simulink model "ADAS_System"  (R2025b)
settings: Solver=FixedStepAuto  StartTime=0.0  StopTime=15  FixedStep=0.01  RelTol=1e-3
values from neighbouring files (symbols this model uses):
  d_init = 160    [init_ADAS.m]
  fs = 100    [init_ADAS.m]
  v_ego = 40    [init_ADAS.m]
  v_lead = 25    [init_ADAS.m]
libraries: simulink x2
settings Model: Creator=szymo  LastModifiedBy=Janek

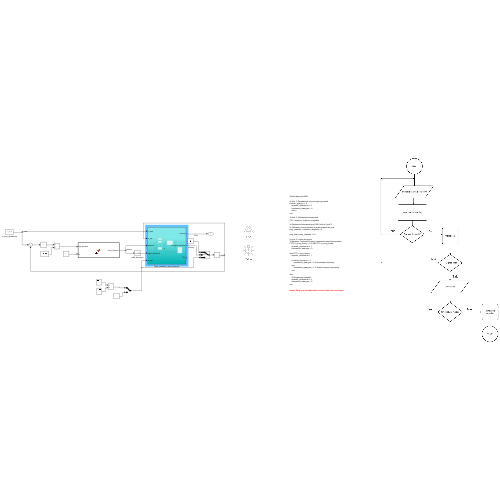
[thumbnail: Simulink's stored preview of the top-level diagram]
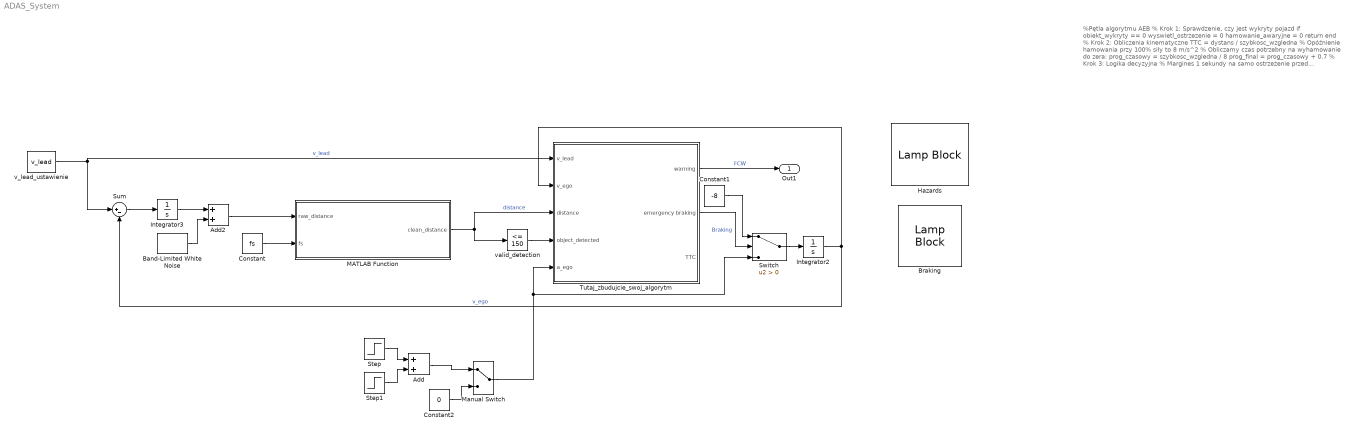
== system ADAS_System ==
  note: %Pętla algorytmu AEB
      |
      | % Krok 1: Sprawdzenie, czy jest wykryty pojazd
      | if obiekt_wykryty == 0
      | wyswietl_ostrzezenie = 0
      | hamowanie_awaryjne = 0
      | return
      | end
      |
      | % Krok 2: Obliczenia kinematyczne
      | TTC = dystans / szybkosc_wzgledna
      |
      | % Opóźnienie hamowania przy 100% siły to 8 m/s^2
      | % Obliczamy czas potrzebny na wyhamowanie do zera:
      | prog_czasowy = szybkosc_wzgledna / 8
      |
      | prog_final = prog_czasowy + 0.7
      |
      | % Krok 3: Logika decyzyjna
      | % Margines 1 sekundy na samo ostrzeżenie przed hamowaniem
      | if TTC < (prog_finalny + 1.0) AND TTC >= prog_finalny
      | wyswietl_ostrzezenie = 1
      | hamowanie_awaryjne = 0
      |
      | elseif TTC < prog_finalny
      | wyswietl_ostrzezenie = 1
      |
      | if reakcja_kierowcy == 1
      | hamowanie_awaryjne = 0 % Hamowanie kierowcy
      | else
      | hamowanie_awaryjne = 1 % System hamuje z pełną siłą
      | end
      |
      | else
      | % Bezpieczna odległość
      | wyswietl_ostrzezenie = 0
      | hamowanie_awaryjne = 0
      | end
      |
      | Uwagi: Zmiany w pseudokodzie oznaczać kolorem czerwonym
  Add : Sum
  Add2 : Sum
  Band-Limited White Noise : simulink/Sources/Band-Limited White Noise  Cov=[0.1]  Ts=0.1  seed=[23341]
  Braking : LampBlock  LabelPosition=Bottom  DefaultColor=[192.0, 192.0, 192.0]  Icon=ExteriorBulbFailure
  Constant : Constant  Value=fs
  Constant1 : Constant  Value=-8
  Constant2 : Constant  Value=0
  Hazards : LampBlock  LabelPosition=Bottom  DefaultColor=[192.0, 192.0, 192.0]  Icon=Hazards
  Integrator2 : Integrator  InitialCondition=v_ego
  Integrator3 : Integrator  InitialCondition=d_init
  MATLAB Function : MATLAB Function  TreatAsAtomicUnit=on
  Manual Switch : ManualSwitch
  Step : Step  Time=8.0  After=-8  SampleTime=0
  Step1 : Step  Time=8.1  After=3  SampleTime=0
  Sum : Sum  Inputs=|+-
  Switch : Switch  Criteria=u2 > Threshold  SaturateOnIntegerOverflow=off  InputSameDT=off
  Tutaj_zbudujcie_swoj_algorytm : Subsystem
  v_lead_ustawienie : Constant  Value=v_lead
  valid_detection : simulink/Logic and Bit Operations/Compare To Constant  relop=<=  const=150  OutDataTypeStr=boolean
  Out1 : Outport
  wires:
  Band-Limited White Noise/1 -> Add2/2
  Add2/1 -> MATLAB Function/1(raw_distance)
  Constant/1 -> MATLAB Function/2(fs)
  Switch/1 -> Integrator2/1
  Integrator2/1 -> Tutaj_zbudujcie_swoj_algorytm/2(v_ego), Sum/2  "v_ego"
  v_lead_ustawienie/1 -> Sum/1, Tutaj_zbudujcie_swoj_algorytm/1(v_lead)  "v_lead"
  Sum/1 -> Integrator3/1
  Integrator3/1 -> Add2/1
  MATLAB Function/1(clean_distance) -> valid_detection/1, Tutaj_zbudujcie_swoj_algorytm/3(distance)  "distance"
  valid_detection/1 -> Tutaj_zbudujcie_swoj_algorytm/4(object_detected)
  Tutaj_zbudujcie_swoj_algorytm/1(warning) -> Out1/1  "FCW"
  Manual Switch/1 -> Tutaj_zbudujcie_swoj_algorytm/5(a_ego), Switch/3
  Constant1/1 -> Switch/1
  Tutaj_zbudujcie_swoj_algorytm/2(emergency braking) -> Switch/2  "Braking"
  Step/1 -> Add/1
  Step1/1 -> Add/2
  Add/1 -> Manual Switch/1
  Constant2/1 -> Manual Switch/2

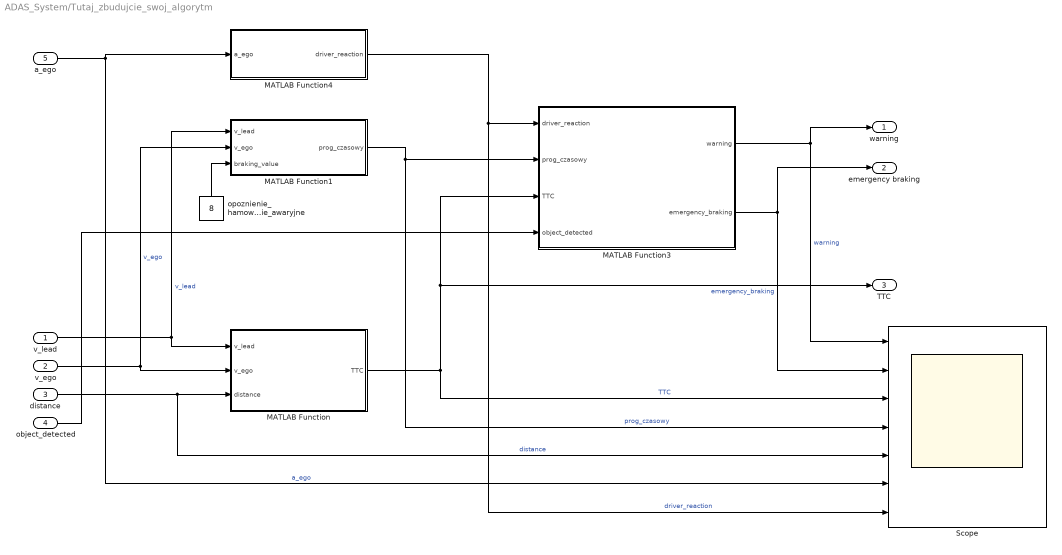
== system ADAS_System/Tutaj_zbudujcie_swoj_algorytm ==
  v_lead : Inport
  v_ego : Inport  Port=2
  distance : Inport  Port=3
  object_detected : Inport  Port=4
  a_ego : Inport  Port=5
  MATLAB Function : MATLAB Function  TreatAsAtomicUnit=on
  MATLAB Function1 : MATLAB Function  TreatAsAtomicUnit=on
  MATLAB Function3 : MATLAB Function  TreatAsAtomicUnit=on
  MATLAB Function4 : MATLAB Function  TreatAsAtomicUnit=on
  Scope : Scope  NumInputPorts=7
      settings: ActiveDisplayYMinimum=146.60609741255024  ActiveDisplayYMaximum=156.61068554348952
  opoznienie_hamowanie_awaryjne : Constant  Value=8
  warning : Outport
  emergency braking : Outport  Port=2
  "TTC " : Outport  Port=3
  wires:
  object_detected/1 -> MATLAB Function3/4(object_detected)
  MATLAB Function3/2(emergency_braking) -> emergency braking/1, Scope/2  "emergency_braking"
  MATLAB Function1/1(prog_czasowy) -> Scope/4, MATLAB Function3/2(prog_czasowy)  "prog_czasowy"
  MATLAB Function/1(TTC) -> MATLAB Function3/3(TTC), "TTC "/1, Scope/3  "TTC"
  v_lead/1 -> MATLAB Function1/1(v_lead), MATLAB Function/1(v_lead)  "v_lead"
  opoznienie_hamowanie_awaryjne/1 -> MATLAB Function1/3(braking_value)
  MATLAB Function3/1(warning) -> warning/1, Scope/1  "warning"
  v_ego/1 -> MATLAB Function1/2(v_ego), MATLAB Function/2(v_ego)  "v_ego"
  distance/1 -> MATLAB Function/3(distance), Scope/5  "distance"
  a_ego/1 -> Scope/6, MATLAB Function4/1(a_ego)  "a_ego"
  MATLAB Function4/1(driver_reaction) -> Scope/7, MATLAB Function3/1(driver_reaction)  "driver_reaction"

== matlab function ADAS_System/Tutaj_zbudujcie_swoj_algorytm/MATLAB Function ==
  data: v_lead input; TTC output; v_ego input; distance input
function TTC = calculate_TTC(v_lead, v_ego, distance)
    delta_v = v_ego - v_lead;
    if delta_v <= 0
        TTC = inf;
    else
        TTC = distance / delta_v;
    end
end

== matlab function ADAS_System/MATLAB Function ==
  settings: updateMethod=DISCRETE
  data: raw_distance input; clean_distance output; fs input
function clean_distance = radar_filter(raw_distance, fs)
    persistent last_dist;
    
    % Inicjalizacja przy pierwszym kroku symulacji
    if isempty(last_dist)
        last_dist = raw_distance;
    end  
    
    % Obliczenie kroku czasu na podstawie częstotliwości próbkowania
    dt = 1 / fs; 
    
    tau = 0.02; 
    
    % Dynamiczne obliczenie wagi dla nowego pomiaru
    alpha = dt / (tau + dt); 
    
    % Filtracja: waga_nowego * nowy_pomiar + waga_starego * stary_pomiar
    clean_distance = alpha * raw_distance + (1 - alpha) * last_dist;
    
    % Zapisanie obecnej wartości na potrzeby kolejnego kroku
    last_dist = clean_distance;
end

== matlab function ADAS_System/Tutaj_zbudujcie_swoj_algorytm/MATLAB Function1 ==
  data: v_lead input; prog_czasowy output; v_ego input; braking_value input
function prog_czasowy = calculate_prog_czasowy(v_lead, v_ego, braking_value)
    delta_v = v_ego - v_lead;
    if delta_v <= 0
        prog_czasowy = inf;
    else
        prog_czasowy = delta_v / braking_value;
    end
end

== matlab function ADAS_System/Tutaj_zbudujcie_swoj_algorytm/MATLAB Function3 ==
  settings: updateMethod=DISCRETE
  data: driver_reaction input; prog_czasowy input; warning output; TTC input; object_detected input; emergency_braking output
function [warning, emergency_braking] = signals_switch(driver_reaction, prog_czasowy, TTC, object_detected)

    persistent is_breaking;
    
    if isempty(is_breaking)
        is_breaking = 0;
    end

    if(TTC < prog_czasowy + 1.7 || is_breaking)
        warning = 1;
    else
        warning = 0;
    end
    
    if(TTC < prog_czasowy + 0.3)
        emergency_braking = 1;
        is_breaking = 1;
        return
    end
    
    if(is_breaking == 1)
        if(isinf(TTC) || driver_reaction)
            emergency_braking = 0;
        else
            emergency_braking = 1;
        end
    else
        if(object_detected && TTC < prog_czasowy + 0.7 && ~driver_reaction)
            emergency_braking = 1;
        else
            emergency_braking = 0;
        end
    end

    is_breaking = emergency_braking;

end

== matlab function ADAS_System/Tutaj_zbudujcie_swoj_algorytm/MATLAB Function4 ==
  settings: updateMethod=DISCRETE
  data: a_ego input; driver_reaction output
function driver_reaction = driver_reaction(a_ego)

    persistent state;

    if isempty(state)
        state = 0;
    end

    if(state == 0)
        if(a_ego < -7)
            driver_reaction = 1;
        else
            driver_reaction = 0;
        end
    else
        if(a_ego > -4)
            driver_reaction = 0;
        else
            driver_reaction = 1;
        end
    end

    state = driver_reaction;

end
